simulink model "py_ma"  (R2021b)
settings: Solver=ode4  StartTime=0.0  StopTime=10.0  FixedStep=1e-3  RelTol=1e-3
settings Model: Creator=Mando  LastModifiedBy=Mando

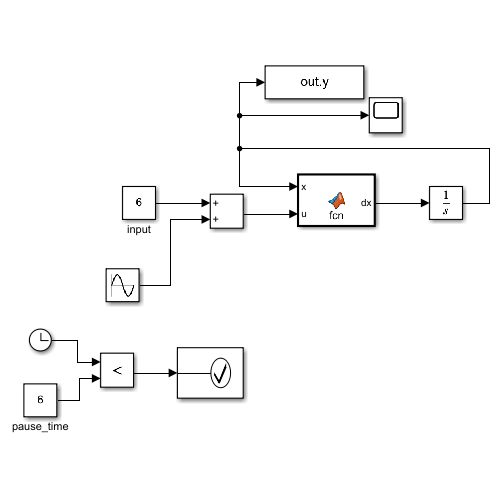
[thumbnail: Simulink's stored preview of the top-level diagram]
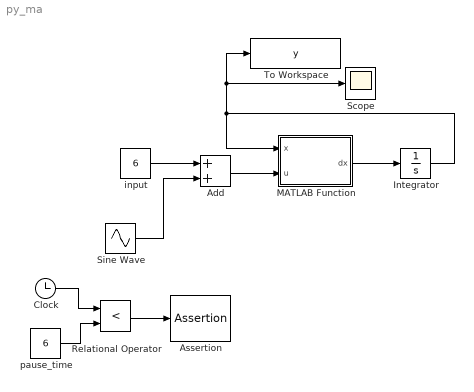
== system py_ma ==
  Add : Sum
  Assertion : Assertion  AssertionFailFcn=set_param(bdroot,'SimulationCommand','pause');  StopWhenAssertionFail=off
  Clock : Clock
  Integrator : Integrator
  MATLAB Function : MATLAB Function  TreatAsAtomicUnit=on
  Relational Operator : RelationalOperator  Operator=<  OutDataTypeStr=boolean  RndMeth=Simplest
  Scope : Scope
  Sine Wave : Sin  Frequency=2*pi*1  SampleTime=0
  To Workspace : ToWorkspace  VariableName=y  SaveFormat=Timeseries  SampleTime=-1
  input : Constant  Value=6
  pause_time : Constant  Value=6
  wires:
  MATLAB Function/1(dx) -> Integrator/1
  Add/1 -> MATLAB Function/2(u)
  Sine Wave/1 -> Add/2
  Integrator/1 -> Scope/1, To Workspace/1, MATLAB Function/1(x)
  input/1 -> Add/1
  pause_time/1 -> Relational Operator/2
  Relational Operator/1 -> Assertion/1
  Clock/1 -> Relational Operator/1

== matlab function py_ma/MATLAB Function ==
  data: x input; u input; dx output
function dx = fcn(x,u)
dx=x+2*u;
